simulink model "Model_FC_v16_Edit_for_Full_Scale_Fuel_Cell_GAS"  (R2018a)
settings: Solver=VariableStepAuto  StartTime=0  StopTime=inf  FixedStep=0.01  RelTol=1e-3  EnableMultiTasking=on
undefined symbols (not defined in the file): sigbuilder_block
libraries: fl_lib x8, simulink x6, nesl_utility x4, autolibdcdc x1, powerlib x1
(part 3 of 3)

== system Model_FC_v16_Edit_for_Full_Scale_Fuel_Cell_GAS/Load ==
  note: This Block models the Load Profile as dictated by the ship Resistance in the River Nile
  Signal : Inport
  Bus Selector : BusSelector  OutputSignals=Cell Output Voltage (V),Number Of Cells
  Current from Load profile of one day : Subsystem  Tag=STV Subsys  LoadFcn=sigbuilder_block('load');  StartFcn=sigbuilder_block('start');  StopFcn=sigbuilder_block('stop');  ClipboardFcn=sigbuilder_block('clipboard');  mask(Sigbuilder block){tuvar=[0:10]}
      mask help: Simulink:masks:SigbuilderBlock_MD
      mask init:
      | if ~strcmp(get_param(bdroot(gcbh),'SimulationStatus'),'stopped') tuvar = sigbuilder_block('maskInit'); end
      settings: CopyFcn=sigbuilder_block('copy');  DeleteFcn=sigbuilder_block('delete');  ModelCloseFcn=sigbuilder_block('modelClose');  PreSaveFcn=sigbuilder_block('preSave');  PauseFcn=sigbuilder_block('pause');  ContinueFcn=sigbuilder_block('continue');  NameChangeFcn=sigbuilder_block('namechange');  OpenFcn=sigbuilder_block('open',[403.5 117 550.5 359.25 ]);  CloseFcn=sigbuilder_block('close');
      mask Display: plot(0, 0, 100, 100,[2, 2, 32, 32, 2], [68, 8, 8, 68, 68],[32, 2], [38, 38], [32, 19, 2],[53, 60, 44], [32, 17, 17, 2],[16, 16, 31, 31]);txt = getActiveGroup(gcbh);text(2, 100, txt,'verticalAlignment', 'top');
  Product : Product
  Terminator : Terminator
  Load Profile Current : Outport
  Total Output Voltage (V) : Outport  Port=2
  wires:
  Signal/1 -> Bus Selector/1
  Bus Selector/1 -> Product/1  "<Cell Output Voltage (V)>"
  Product/1 -> Total Output Voltage (V)/1  "Total Output Voltage (V)"
  Current from Load profile of one day/2(Signal 2) -> Load Profile Current/1  "Current from Load profile (Alex to Aswan)"
  Bus Selector/2 -> Product/2  "<Number Of Cells>"
  Current from Load profile of one day/1(Signal 1) -> Terminator/1  "Current from Load profile (Alex to Aswan)"

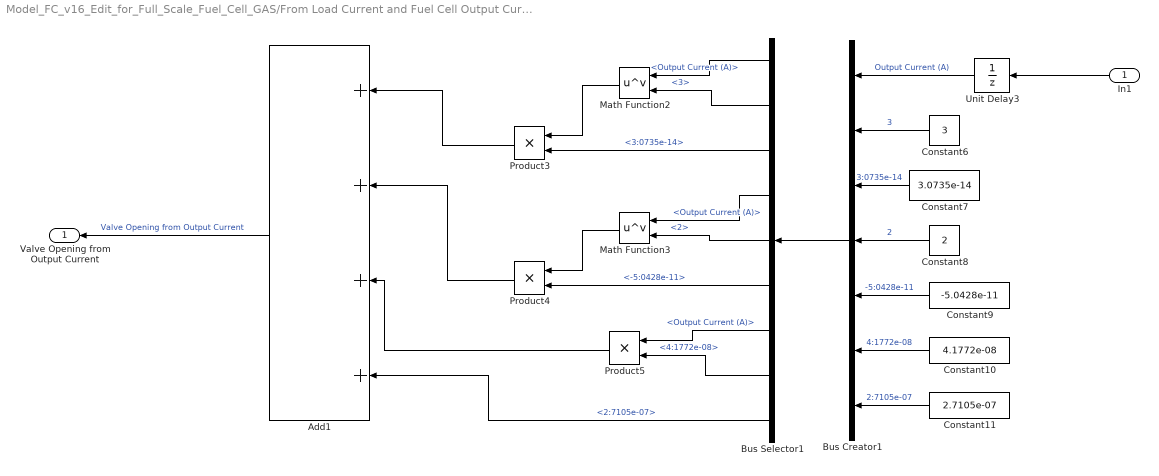
== system Model_FC_v16_Edit_for_Full_Scale_Fuel_Cell_GAS/From Load Current and Fuel Cell Output Current (A) to Valve Restriction Area (m^2)/Subsystem ==
  In1 : Inport
  Add1 : Sum  Inputs=4
  Bus Creator1 : BusCreator  Inputs=7
  Bus Selector1 : BusSelector  OutputSignals=Output Current (A),3,3:0735e-14,Output Current (A),2,-5:0428e-11,Output Current (A),4:1772e-08,2:7105e-07
  Constant10 : Constant  Value=4.1772e-08
  Constant11 : Constant  Value=2.7105e-07
  Constant6 : Constant  Value=3
  Constant7 : Constant  Value=3.0735e-14
  Constant8 : Constant  Value=2
  Constant9 : Constant  Value=-5.0428e-11
  Math Function2 : Math  Operator=pow  SaturateOnIntegerOverflow=on
  Math Function3 : Math  Operator=pow  SaturateOnIntegerOverflow=on
  Product3 : Product
  Product4 : Product
  Product5 : Product
  Unit Delay3 : UnitDelay  SampleTime=-1
  Valve Opening from Output Current : Outport
  wires:
  Product3/1 -> Add1/1
  Constant9/1 -> Bus Creator1/5  "-5:0428e-11"
  Constant11/1 -> Bus Creator1/7  "2:7105e-07"
  Constant8/1 -> Bus Creator1/4  "2"
  Constant6/1 -> Bus Creator1/2  "3"
  Bus Selector1/5 -> Math Function3/2  "<2>"
  Constant10/1 -> Bus Creator1/6  "4:1772e-08"
  In1/1 -> Unit Delay3/1
  Math Function2/1 -> Product3/1
  Math Function3/1 -> Product4/1
  Bus Selector1/3 -> Product3/2  "<3:0735e-14>"
  Bus Selector1/9 -> Add1/4  "<2:7105e-07>"
  Bus Selector1/2 -> Math Function2/2  "<3>"
  Bus Creator1/1 -> Bus Selector1/1
  Bus Selector1/6 -> Product4/2  "<-5:0428e-11>"
  Bus Selector1/8 -> Product5/2  "<4:1772e-08>"
  Bus Selector1/4 -> Math Function3/1  "<Output Current (A)>"
  Product4/1 -> Add1/2
  Product5/1 -> Add1/3
  Constant7/1 -> Bus Creator1/3  "3:0735e-14"
  Unit Delay3/1 -> Bus Creator1/1  "Output Current (A)"
  Bus Selector1/7 -> Product5/1  "<Output Current (A)>"
  Bus Selector1/1 -> Math Function2/1  "<Output Current (A)>"
  Add1/1 -> Valve Opening from Output Current/1  "Valve Opening from Output Current"

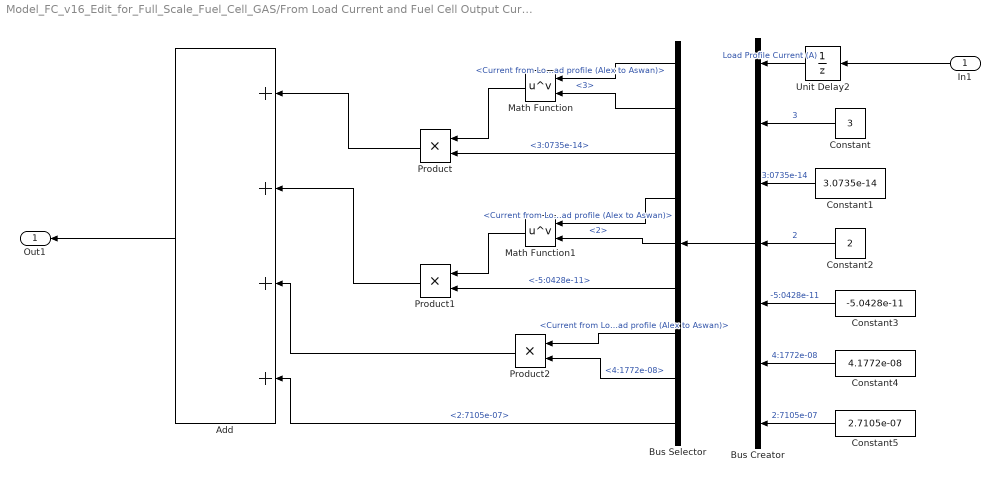
== system Model_FC_v16_Edit_for_Full_Scale_Fuel_Cell_GAS/From Load Current and Fuel Cell Output Current (A) to Valve Restriction Area (m^2)/Subsystem1 ==
  In1 : Inport
  Add : Sum  Inputs=4
  Bus Creator : BusCreator  Inputs=7
  Bus Selector : BusSelector  OutputSignals=Load Profile Current (A).Current from Load profile (Alex to Aswan),3,3:0735e-14,Load Profile Current (A).Current from Load profile (Alex to Aswan),2,-5:0428e-11,Load Profile Current (A).Current from Load profile (Alex to Aswan),4:1772e-08,2:7105e-07
  Constant : Constant  Value=3
  Constant1 : Constant  Value=3.0735e-14
  Constant2 : Constant  Value=2
  Constant3 : Constant  Value=-5.0428e-11
  Constant4 : Constant  Value=4.1772e-08
  Constant5 : Constant  Value=2.7105e-07
  Math Function : Math  Operator=pow  SaturateOnIntegerOverflow=on
  Math Function1 : Math  Operator=pow  SaturateOnIntegerOverflow=on
  Product : Product
  Product1 : Product
  Product2 : Product
  Unit Delay2 : UnitDelay  SampleTime=-1
  Out1 : Outport
  wires:
  Bus Selector/2 -> Math Function/2  "<3>"
  Bus Selector/5 -> Math Function1/2  "<2>"
  Product/1 -> Add/1
  Constant/1 -> Bus Creator/2  "3"
  Unit Delay2/1 -> Bus Creator/1  "Load Profile Current (A)"
  Constant5/1 -> Bus Creator/7  "2:7105e-07"
  Constant2/1 -> Bus Creator/4  "2"
  Bus Selector/1 -> Math Function/1  "<Current from Load profile (Alex to Aswan)>"
  Constant3/1 -> Bus Creator/5  "-5:0428e-11"
  Constant4/1 -> Bus Creator/6  "4:1772e-08"
  Bus Selector/7 -> Product2/1  "<Current from Load profile (Alex to Aswan)>"
  Math Function1/1 -> Product1/1
  Bus Selector/9 -> Add/4  "<2:7105e-07>"
  Bus Selector/8 -> Product2/2  "<4:1772e-08>"
  Bus Selector/6 -> Product1/2  "<-5:0428e-11>"
  Constant1/1 -> Bus Creator/3  "3:0735e-14"
  Product1/1 -> Add/2
  Math Function/1 -> Product/1
  Bus Creator/1 -> Bus Selector/1
  Product2/1 -> Add/3
  Bus Selector/3 -> Product/2  "<3:0735e-14>"
  Bus Selector/4 -> Math Function1/1  "<Current from Load profile (Alex to Aswan)>"
  In1/1 -> Unit Delay2/1
  Add/1 -> Out1/1

== system Model_FC_v16_Edit_for_Full_Scale_Fuel_Cell_GAS/Fuel Cell Model/ From Current Density (A//cm^2) To Overvoltages (V) ==
  note: This Block calculates all the Resistances in the Fuel Cell
      | 1-Activation Overvoltage 2- Ohmic Overvoltage 3-Concentration Overvoltage
      | INPUTS: INPUTS: A) Current Density (A/cm^2) INPUTS: A) Current Density (A/cm^2)
      | A) Current Density (A/cm^2) OUTPUTS: A) Ohmic Overvoltage (V) OUTPUTS: A) Concentration Overvoltage (V)
      | B) Temperature (c)
      |
      | OUTPUTS:
      | A) Activation Overvoltage (V)
  Current Density (A/cm^2) : Inport
  Temperature (C) : Inport  Port=2
  Activation Overvoltage : Subsystem
  Concentration Overvoltage : Subsystem
  Ohmic Overvoltage : Subsystem
  Activation Overvoltage (V) : Outport
  Ohmic Overvoltage (V) : Outport  Port=2
  Concentration Overvoltage (V) : Outport  Port=3
  Exchange Current Density (i_0) : Outport  Port=4
  wires:
  Temperature (C)/1 -> Activation Overvoltage/1(Temperature/C1)
  Current Density (A/cm^2)/1 -> Activation Overvoltage/2(Current Density (i)(A/cm^2)), Concentration Overvoltage/1(Current Density (i)1), Ohmic Overvoltage/1(Current Density (i ))
  Ohmic Overvoltage/1(V_Resistive) -> Ohmic Overvoltage (V)/1
  Activation Overvoltage/1(Activation Overvoltage1 (V)) -> Activation Overvoltage (V)/1
  Concentration Overvoltage/1("Concentration Overvoltage1 (V) ") -> Concentration Overvoltage (V)/1
  Activation Overvoltage/2(Exchange Current Density (i_0)) -> Exchange Current Density (i_0)/1

== system Model_FC_v16_Edit_for_Full_Scale_Fuel_Cell_GAS/Fuel Cell Model/Air Flow Rate To Current (A) ==
  note: The function of this block is: To calculate the Air Mass Flow Rate in (kg/s) using the Input Current Density (A/cm^2)
      | Inputs: Outputs:
      | a) Current DEnsity (A/cm^2) A) Air Mass Flow Rate (kg/s)
      | b) Cell Area (cm^2)
      | c) Number of Cells
  Current Density (A/cm^2) : Inport
  Cell Area (cm^2) : Inport  Port=2
  Number Of Cells : Inport  Port=3
  Air Molar Mass (Kg) : Constant  Value=28.9647e-3
  Current (A) : Product
  Divide : Product  Inputs=*/
  From Stack Current (A) To Oxygen Mass Flow Rate(kg/s) : Subsystem
  Oxygen Molar Mass per One Mole of Air (Kg) : Constant  Value=6.72e-3
  Product : Product
  Air Mass Flow Rate (kg/s) : Outport
  wires:
  Current (A)/1 -> From Stack Current (A) To Oxygen Mass Flow Rate(kg/s)/1(Current (A))
  Number Of Cells/1 -> From Stack Current (A) To Oxygen Mass Flow Rate(kg/s)/2(Number Of Cells)
  From Stack Current (A) To Oxygen Mass Flow Rate(kg/s)/1(Oxygen Flow Rate (kg/s)) -> Product/1
  Current Density (A/cm^2)/1 -> Current (A)/1
  Cell Area (cm^2)/1 -> Current (A)/2
  Air Molar Mass (Kg)/1 -> Product/2
  Product/1 -> Divide/1
  Oxygen Molar Mass per One Mole of Air (Kg)/1 -> Divide/2
  Divide/1 -> Air Mass Flow Rate (kg/s)/1  "Air Mass Flow Rate (kg/s)"

== system Model_FC_v16_Edit_for_Full_Scale_Fuel_Cell_GAS/Fuel Cell Model/Current Density A//cm^2 (Polarization Curve) ==
  Demux : Demux  Tag=STV Demux  Outputs=2
  FromWs : FromWorkspace  Tag=STV FromWs  VariableName=tuvar  SampleTime=0
      SigBuilderData=|
      | common.afterFinalStr = 'Extrapolate'
      | common.sampleTime = 0
      | dataSet.timeRange = [0 20]
      | dataSet.name = 'Group 1'
      | sbobj.Groups.Name = 'Group 1'
      | sbobj.Groups.Signals(1).Name = 'Signal 1'
      | sbobj.Groups.Signals(1).XData = [0 0.5 1 20]
      | sbobj.Groups.Signals(1).YData = [0.01 1 1.4 1.4]
      | sbobj.Groups.Signals(2).Name = 'Signal 2'
      | sbobj.Groups.Signals(2).XData = [0 20]
      | sbobj.Groups.Signals(2).YData = [1 1]
      | sbobj.Groups.TimeRange = [0 20]
  Signal 1 : Outport  Tag=STV Outport
  Signal 2 : Outport  Tag=STV Outport  Port=2
  wires:
  Demux/1 -> Signal 1/1
  FromWs/1 -> Demux/1
  Demux/2 -> Signal 2/1

== system Model_FC_v16_Edit_for_Full_Scale_Fuel_Cell_GAS/Fuel Cell Model/From Mass Flow Rates (kg//s) To Current Density (A//cm^2) ==
  note: The function of this block is to convert the input Hydrogen Mass Flow rate (Kg/s) to Current (A) then divide it by the Cell Area (cm^2) to get (Current Density) (A/cm^2)
      | which will be the input of several other blocks.
      | Inputs: a)Hydrogen Mass Flow Rate (kg/s) Outputs: Current Density (A/cm^2)
      | b)Number of Cells
      | c) Cell Area (cm^2)
  Hydrogen Flow Rate (kg/s) : Inport
  Cell Area (cm^2) : Inport  Port=2
  Number Of Cells : Inport  Port=3
  From Current (A) To Current Density (A/cm^2) : Subsystem
  Fuel Mass Flow Rate (kg/s) To Current (A) : Subsystem
  Current Density (A/cm^2) : Outport
  wires:
  Cell Area (cm^2)/1 -> From Current (A) To Current Density (A/cm^2)/2(Cell Area (cm^2))
  Fuel Mass Flow Rate (kg/s) To Current (A)/1(Current (A)) -> From Current (A) To Current Density (A/cm^2)/1(Nominal Current (A))
  Hydrogen Flow Rate (kg/s)/1 -> Fuel Mass Flow Rate (kg/s) To Current (A)/1(Hydrogen Flow Rate (kg/s))
  From Current (A) To Current Density (A/cm^2)/1(Current Density (A/cm^2)) -> Current Density (A/cm^2)/1  "Current density (A/cm^2)"
  Number Of Cells/1 -> Fuel Mass Flow Rate (kg/s) To Current (A)/2(Number Of Cells)  "Number Of Cells"

== system Model_FC_v16_Edit_for_Full_Scale_Fuel_Cell_GAS/Fuel Cell Model/From Pressures (atm) To Nernest Voltage (V) ==
  note: This Block calculates the Partial Pressures of Hydrogen and Oxygen (atm) from their pressures (atm) then uses these values to calculate the Nernest Voltage (V)
      |
      | INPUTS: A) Current Density (i) (A/cm^2) OUTPUTS 1: A) Oxygen Partial Pressure (atm) OUTPUTS 2: A) Nernest Voltage (V)
      | B) Absolute Hydrogen Pressure (atm) B) Water Saturation Pressure (atm)
      | C) Absolute Air Pressure (atm) C) Hydrogen Partial Pressure(atm)
      | D) Temperature (c)
  Current Density (i) : Inport
  Hydrogen Pressure (atm) : Inport  Port=2
  Air Pressure (atm) : Inport  Port=3
  Temperature (C) : Inport  Port=4
  From Absolute Pressure (atm) To Partial Pressures (atm) : Subsystem
  From Partial Pressures (atm) To Nernest Voltage (V) : Subsystem
  Oxygen Partial Pressure : Outport
  Nernest Voltage (V) : Outport  Port=2
  Water Pressure : Outport  Port=3
  wires:
  Temperature (C)/1 -> From Partial Pressures (atm) To Nernest Voltage (V)/4(Temperature/C), From Absolute Pressure (atm) To Partial Pressures (atm)/4(Temperature/C)
  From Absolute Pressure (atm) To Partial Pressures (atm)/1(Hydrogen Partial Pressure (pp_H2)) -> From Partial Pressures (atm) To Nernest Voltage (V)/1(Hydrogen Partial Pressure)
  Hydrogen Pressure (atm)/1 -> From Absolute Pressure (atm) To Partial Pressures (atm)/2(Hydrogen Pressure (P_H2))
  From Partial Pressures (atm) To Nernest Voltage (V)/1(Nernest Voltage1) -> Nernest Voltage (V)/1
  From Absolute Pressure (atm) To Partial Pressures (atm)/2(Oxygen Partial Pressure pp_O2) -> Oxygen Partial Pressure/1, From Partial Pressures (atm) To Nernest Voltage (V)/2(Oxygen Partial Pressure)
  From Absolute Pressure (atm) To Partial Pressures (atm)/3(Water Pressure) -> Water Pressure/1, From Partial Pressures (atm) To Nernest Voltage (V)/3(Water Pressure (P_H2O))
  Current Density (i)/1 -> From Absolute Pressure (atm) To Partial Pressures (atm)/1(Current Density (i ))
  Air Pressure (atm)/1 -> From Absolute Pressure (atm) To Partial Pressures (atm)/3(Air Pressure (P_air))

== system Model_FC_v16_Edit_for_Full_Scale_Fuel_Cell_GAS/Load/Current from Load profile of one day ==
  Demux : Demux  Tag=STV Demux  Outputs=2
  FromWs : FromWorkspace  Tag=STV FromWs  VariableName=tuvar  SampleTime=0
      SigBuilderData=|
      | common.afterFinalStr = 'Extrapolate'
      | common.sampleTime = 0
      | dataSet.timeRange = [0 300]
      | dataSet.name = 'Group 1'
      | sbobj.Groups.Name = 'Group 1'
      | sbobj.Groups.Signals(1).Name = 'Signal 1'
      | sbobj.Groups.Signals(1).XData = [0 2.75 2.75 5.75 5.75 10.98 10.98 24 24 24.6 24.6 27.61 27.61 30.61 30.61 33.73 33.73 36.73 48 48 52.19 52.19 55.19 55.19 59.38 59.38 62.38 72 72 84 84 96 96 108 108 120 120 132 132 144 144 146.76 146.76 147.76 147.76 156 156 168 168 175.76 175.76 176.76 176.76 180 180 192 192 204 204 216 216 216.76 216.76 217.76 217.76 228 228 240 240 244.83 244.83 300]
      | sbobj.Groups.Signals(1).YData = [145.4545455 145.4545455 0.01 0.01 145.4545455 145.4545455 0.01 0.01 195.4545455 195.4545455 486.3636364 486.3636364 0.01 0.01 404.5454545 404.5454545 0.01 0.01 0.01 486.3636364 486.3636364 0.01 0.01 486.3636364 486.3636364 0.01 0.01 0.01 463.6363636 463.6363636 0.01 0.01 463.6363636 463.6363636 0.01 0.01 463.6363636 463.6363636 0.01 0.01 463.6363636 463.6363636 0.01 0.01 463.6363636 463.6363636 0.01 0.01 463.6363636 463.6363636 0.01 0.01 463.6363636 463.6363636 0.01 0.01 463.6363636 463.6363636 0.01 0.01 463.6363636 463.6363636 0.01 0.01 463.6363636 463.6363636 0.01 0.01 463.6363636 463.6363636 0.01 0.01]
      | sbobj.Groups.Signals(2).Name = 'Signal 2'
      | sbobj.Groups.Signals(2).XData = [0 300]
      | sbobj.Groups.Signals(2).YData = [243 243]
      | sbobj.Groups.TimeRange = [0 300]
  Signal 1 : Outport  Tag=STV Outport
  Signal 2 : Outport  Tag=STV Outport  Port=2
  wires:
  Demux/1 -> Signal 1/1
  FromWs/1 -> Demux/1
  Demux/2 -> Signal 2/1

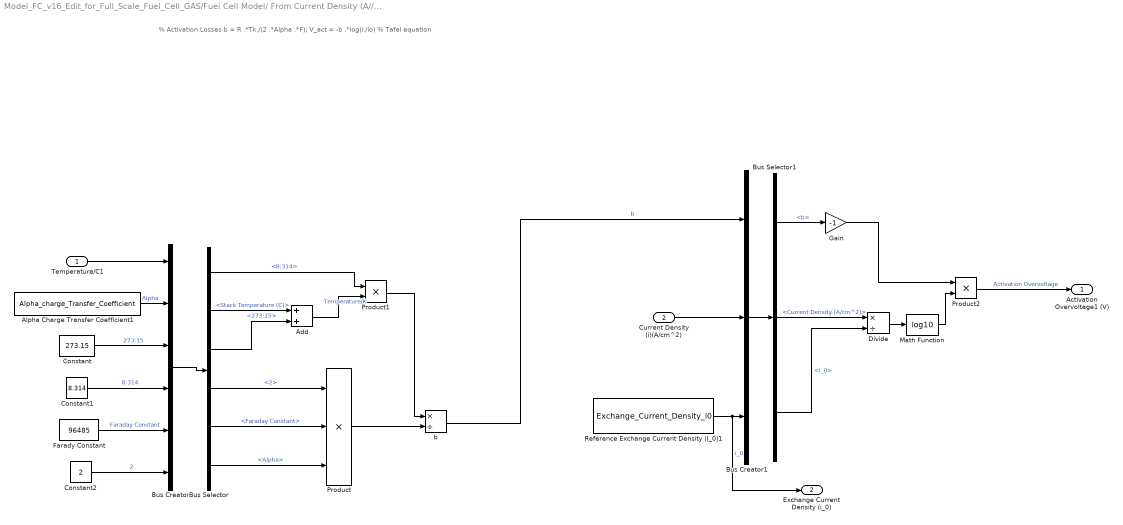
== system Model_FC_v16_Edit_for_Full_Scale_Fuel_Cell_GAS/Fuel Cell Model/ From Current Density (A//cm^2) To Overvoltages (V)/Activation Overvoltage ==
  note: % Activation Losses
      | b = R .*Tk./(2 .*Alpha .*F);
      | V_act = -b .*log(i./io) % Tafel equation
  Temperature/C1 : Inport
  Current Density (i)(A/cm^2) : Inport  Port=2
  Add : Sum
  Alpha Charge Transfer Coefficient1 : Constant  Value=Alpha_charge_Transfer_Coefficient
  Bus Creator : BusCreator  Inputs=6
  Bus Creator1 : BusCreator  Inputs=3
  Bus Selector : BusSelector  OutputSignals=8:314,Stack Temperature (C),273:15,2,Faraday Constant,Alpha
  Bus Selector1 : BusSelector  OutputSignals=b,Current Density (A/cm^2),i_0
  Constant : Constant  Value=273.15
  Constant1 : Constant  Value=8.314
  Constant2 : Constant  Value=2
  Divide : Product  Inputs=*/
  Farady Constant : Constant  Value=96485
  Gain : Gain  Gain=-1
  Math Function : Math  Operator=log10  SaturateOnIntegerOverflow=on
  Product : Product  Inputs=3
  Product1 : Product
  Product2 : Product
  Reference Exchange Current Density (I_0)1 : Constant  Value=Exchange_Current_Density_i0
  b : Product  Inputs=*/
  Activation Overvoltage1 (V) : Outport
  Exchange Current Density (i_0) : Outport  Port=2
  wires:
  Alpha Charge Transfer Coefficient1/1 -> Bus Creator/2  "Alpha"
  Temperature/C1/1 -> Bus Creator/1
  Current Density (i)(A/cm^2)/1 -> Bus Creator1/2
  Reference Exchange Current Density (I_0)1/1 -> Bus Creator1/3, Exchange Current Density (i_0)/1  "i_0"
  Product2/1 -> Activation Overvoltage1 (V)/1  "Activation Overvoltage"
  Bus Creator/1 -> Bus Selector/1
  Constant/1 -> Bus Creator/3  "273:15"
  Constant1/1 -> Bus Creator/4  "8:314"
  Farady Constant/1 -> Bus Creator/5  "Faraday Constant"
  Constant2/1 -> Bus Creator/6  "2"
  Bus Selector/4 -> Product/1  "<2>"
  Bus Selector/5 -> Product/2  "<Faraday Constant>"
  Bus Selector/6 -> Product/3  "<Alpha>"
  Product/1 -> b/2
  Bus Selector/1 -> Product1/1  "<8:314>"
  Bus Selector/2 -> Add/1  "<Stack Temperature (C)>"
  Bus Selector/3 -> Add/2  "<273:15>"
  Add/1 -> Product1/2  "Temperature/K"
  Product1/1 -> b/1
  b/1 -> Bus Creator1/1  "b"
  Bus Creator1/1 -> Bus Selector1/1
  Bus Selector1/1 -> Gain/1  "<b>"
  Bus Selector1/2 -> Divide/1  "<Current Density (A/cm^2)>"
  Bus Selector1/3 -> Divide/2  "<i_0>"
  Gain/1 -> Product2/1
  Divide/1 -> Math Function/1
  Math Function/1 -> Product2/2

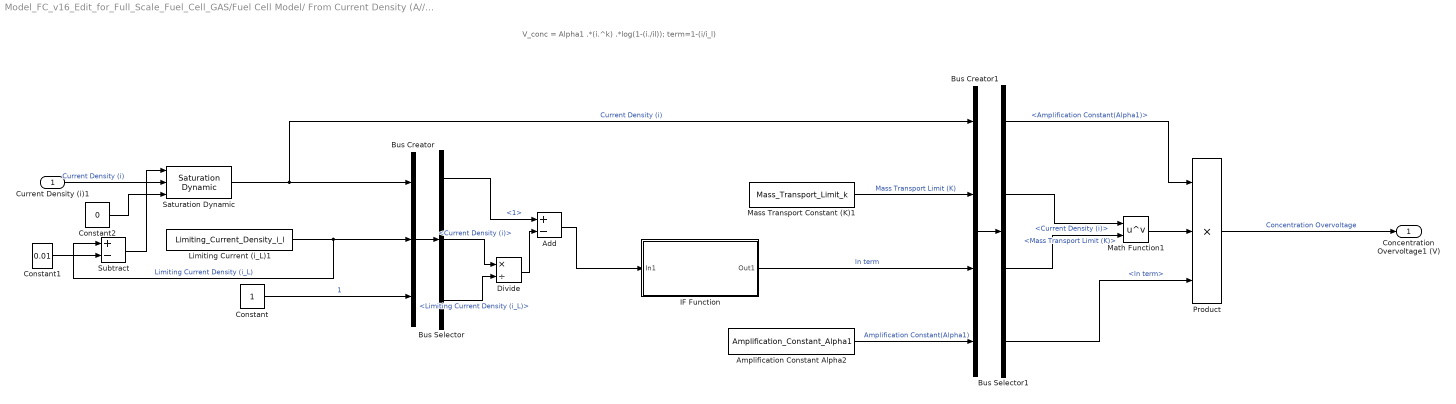
== system Model_FC_v16_Edit_for_Full_Scale_Fuel_Cell_GAS/Fuel Cell Model/ From Current Density (A//cm^2) To Overvoltages (V)/Concentration Overvoltage ==
  note: V_conc = Alpha1 .*(i.^k) .*log(1-(i./il));
      | term=1-(i/i_l)
  Current Density (i)1 : Inport
  Add : Sum  Inputs=+-
  Amplification Constant Alpha2 : Constant  Value=Amplification_Constant_Alpha1
  Bus Creator : BusCreator  Inputs=3
  Bus Creator1 : BusCreator  Inputs=4
  Bus Selector : BusSelector  OutputSignals=1,Current Density (i),Limiting Current Density (i_L)
  Bus Selector1 : BusSelector  OutputSignals=Amplification Constant(Alpha1),Current Density (i),Mass Transport Limit (K),ln term
  Constant : Constant
  Constant1 : Constant  Value=0.01
  Constant2 : Constant  Value=0
  Divide : Product  Inputs=*/
  IF Function : Subsystem
  Limiting Current (i_L)1 : Constant  Value=Limiting_Current_Density_i_l
  Mass Transport Constant (K)1 : Constant  Value=Mass_Transport_Limit_k
  Math Function1 : Math  Operator=pow  SaturateOnIntegerOverflow=on
  Product : Product  Inputs=3
  Saturation Dynamic : simulink/Discontinuities/Saturation Dynamic  OutMin=[]  OutMax=[]  OutDataTypeStr=Inherit: Same as second input  OutDataType=fixdt(1, 16)  OutScaling=2^-10  DoSatur=off
  Subtract : Sum  Inputs=+-
  "Concentration Overvoltage1 (V) " : Outport
  wires:
  Bus Creator/1 -> Bus Selector/1
  Limiting Current (i_L)1/1 -> Subtract/1, Bus Creator/2  "Limiting Current Density (i_L)"
  Saturation Dynamic/1 -> Bus Creator1/1, Bus Creator/1  "Current Density (i)"
  Mass Transport Constant (K)1/1 -> Bus Creator1/2  "Mass Transport Limit (K)"
  Amplification Constant Alpha2/1 -> Bus Creator1/4  "Amplification Constant(Alpha1)"
  Product/1 -> "Concentration Overvoltage1 (V) "/1  "Concentration Overvoltage"
  Constant/1 -> Bus Creator/3  "1"
  Bus Selector/1 -> Add/1  "<1>"
  Bus Selector/2 -> Divide/1  "<Current Density (i)>"
  Bus Selector/3 -> Divide/2  "<Limiting Current Density (i_L)>"
  Divide/1 -> Add/2
  Add/1 -> IF Function/1(In1)
  IF Function/1(Out1) -> Bus Creator1/3  "ln term"
  Bus Creator1/1 -> Bus Selector1/1
  Bus Selector1/1 -> Product/1  "<Amplification Constant(Alpha1)>"
  Bus Selector1/2 -> Math Function1/1  "<Current Density (i)>"
  Bus Selector1/3 -> Math Function1/2  "<Mass Transport Limit (K)>"
  Bus Selector1/4 -> Product/3  "<ln term>"
  Math Function1/1 -> Product/2
  Current Density (i)1/1 -> Saturation Dynamic/2  "Current Density (i)"
  Constant1/1 -> Subtract/2
  Subtract/1 -> Saturation Dynamic/1
  Constant2/1 -> Saturation Dynamic/3

== system Model_FC_v16_Edit_for_Full_Scale_Fuel_Cell_GAS/Fuel Cell Model/ From Current Density (A//cm^2) To Overvoltages (V)/Ohmic Overvoltage ==
  Current Density (i ) : Inport
  Constant : Constant  Value=-1
  Internal Resistance (r) : Constant  Value=Internal_Resistance_r
  V_Resistive1 : Product  Inputs=3
  V_Resistive : Outport
  wires:
  Constant/1 -> V_Resistive1/3
  Internal Resistance (r)/1 -> V_Resistive1/2
  Current Density (i )/1 -> V_Resistive1/1
  V_Resistive1/1 -> V_Resistive/1  "Ohmic Overvoltage (V)"

== system Model_FC_v16_Edit_for_Full_Scale_Fuel_Cell_GAS/Fuel Cell Model/Air Flow Rate To Current (A)/From Stack Current (A) To Oxygen Mass Flow Rate(kg//s) ==
  Current (A) : Inport
  Number Of Cells : Inport  Port=2
  Divide : Product  Inputs=*/
  F : Constant  Value=96487
  Oxygen Molar Mass (Kg/mol) : Constant  Value=32e-3
  Product : Product
  Product1 : Product
  Product2 : Product
  c : Constant  Value=4
  Oxygen Flow Rate (kg/s) : Outport
  wires:
  F/1 -> Product1/1
  Current (A)/1 -> Product/1
  Product/1 -> Divide/1
  Oxygen Molar Mass (Kg/mol)/1 -> Product2/2
  c/1 -> Product1/2
  Divide/1 -> Product2/1
  Product1/1 -> Divide/2
  Product2/1 -> Oxygen Flow Rate (kg/s)/1
  Number Of Cells/1 -> Product/2

== system Model_FC_v16_Edit_for_Full_Scale_Fuel_Cell_GAS/Fuel Cell Model/From Mass Flow Rates (kg//s) To Current Density (A//cm^2)/From Current (A) To Current Density (A//cm^2) ==
  note: i=I/A
      | where i=Current Density (A/cm^2)
      | I= Current (A)
      | A=Cell Area (cm^2)
  Nominal Current (A) : Inport
  Cell Area (cm^2) : Inport  Port=2
  Divide : Product  Inputs=*/
  Current Density (A/cm^2) : Outport
  wires:
  Nominal Current (A)/1 -> Divide/1
  Cell Area (cm^2)/1 -> Divide/2
  Divide/1 -> Current Density (A/cm^2)/1

== system Model_FC_v16_Edit_for_Full_Scale_Fuel_Cell_GAS/Fuel Cell Model/From Mass Flow Rates (kg//s) To Current Density (A//cm^2)/Fuel Mass Flow Rate (kg//s) To Current (A) ==
  note: This block calculates the output Current (A) from the Hydrogen Mass Flow Rate (kg/s)
      | I=Hydrogen Mass Flow Rate (kg/s)*2*F/(M_H2*n)
      | where: I=Current (A)
      | F=Faraday Constant=96487 C/mol
      | M_H2=hydrogen molar mass=2.016*10^-3 kg/mol
      | n=Number of Cells
  Hydrogen Flow Rate (kg/s) : Inport
  Number Of Cells : Inport  Port=2
  Constant1 : Constant  Value=2
  Divide : Product  Inputs=*/
  F : Constant  Value=96487
  Hydrogen Molar Mass : Constant  Value=2.016e-3
  Product : Product
  Product1 : Product
  Product2 : Product
  Current (A) : Outport
  wires:
  F/1 -> Product1/2
  Constant1/1 -> Product1/1
  Product1/1 -> Product/2
  Product/1 -> Divide/1
  Hydrogen Molar Mass/1 -> Product2/1
  Number Of Cells/1 -> Product2/2
  Product2/1 -> Divide/2
  Divide/1 -> Current (A)/1
  Hydrogen Flow Rate (kg/s)/1 -> Product/1

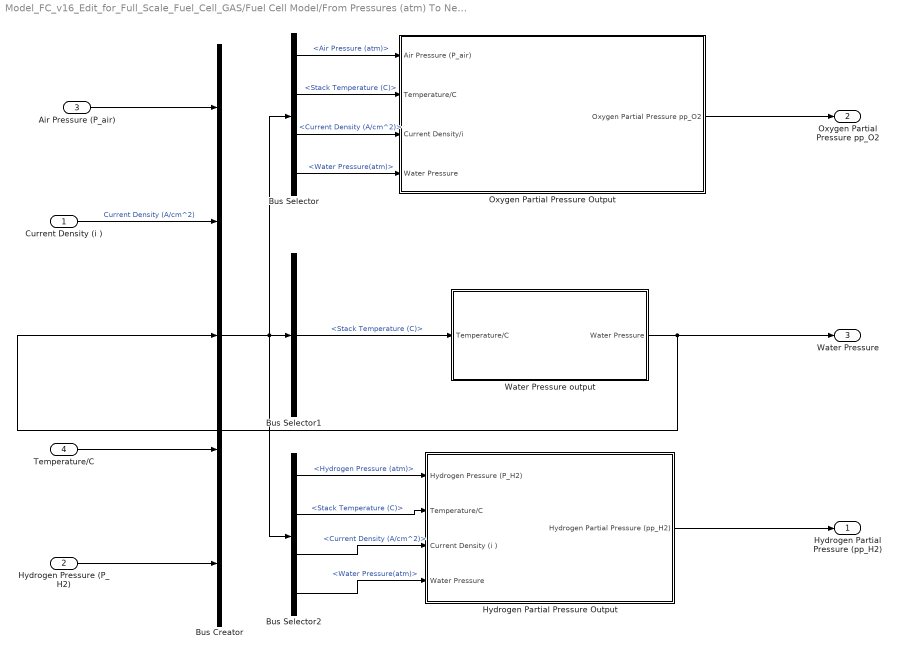
== system Model_FC_v16_Edit_for_Full_Scale_Fuel_Cell_GAS/Fuel Cell Model/From Pressures (atm) To Nernest Voltage (V)/From Absolute Pressure (atm) To Partial Pressures (atm) ==
  Current Density (i ) : Inport
  Hydrogen Pressure (P_H2) : Inport  Port=2
  Air Pressure (P_air) : Inport  Port=3
  Temperature/C : Inport  Port=4
  Bus Creator : BusCreator  Inputs=5
  Bus Selector : BusSelector  OutputSignals=Air Pressure (atm),Stack Temperature (C),Current Density (A/cm^2),Water Pressure(atm)
  Bus Selector1 : BusSelector  OutputSignals=Stack Temperature (C)
  Bus Selector2 : BusSelector  OutputSignals=Hydrogen Pressure (atm),Stack Temperature (C),Current Density (A/cm^2),Water Pressure(atm)
  Hydrogen Partial Pressure Output : Subsystem
  Oxygen Partial Pressure Output : Subsystem
  Water Pressure output : Subsystem
  Hydrogen Partial Pressure (pp_H2) : Outport
  Oxygen Partial Pressure pp_O2 : Outport  Port=2
  Water Pressure : Outport  Port=3
  wires:
  Water Pressure output/1(Water Pressure) -> Water Pressure/1, Bus Creator/3
  Air Pressure (P_air)/1 -> Bus Creator/1
  Oxygen Partial Pressure Output/1(Oxygen Partial Pressure pp_O2) -> Oxygen Partial Pressure pp_O2/1
  Hydrogen Partial Pressure Output/1(Hydrogen Partial Pressure (pp_H2)) -> Hydrogen Partial Pressure (pp_H2)/1
  Current Density (i )/1 -> Bus Creator/2  "Current Density (A/cm^2)"
  Temperature/C/1 -> Bus Creator/4
  Hydrogen Pressure (P_H2)/1 -> Bus Creator/5
  Bus Creator/1 -> Bus Selector2/1, Bus Selector/1, Bus Selector1/1
  Bus Selector/1 -> Oxygen Partial Pressure Output/1(Air Pressure (P_air))  "<Air Pressure (atm)>"
  Bus Selector/2 -> Oxygen Partial Pressure Output/2(Temperature/C)  "<Stack Temperature (C)>"
  Bus Selector/3 -> Oxygen Partial Pressure Output/3(Current Density/i)  "<Current Density (A/cm^2)>"
  Bus Selector/4 -> Oxygen Partial Pressure Output/4(Water Pressure)  "<Water Pressure(atm)>"
  Bus Selector1/1 -> Water Pressure output/1(Temperature/C)  "<Stack Temperature (C)>"
  Bus Selector2/1 -> Hydrogen Partial Pressure Output/1(Hydrogen Pressure (P_H2))  "<Hydrogen Pressure (atm)>"
  Bus Selector2/2 -> Hydrogen Partial Pressure Output/2(Temperature/C)  "<Stack Temperature (C)>"
  Bus Selector2/3 -> Hydrogen Partial Pressure Output/3(Current Density (i ))  "<Current Density (A/cm^2)>"
  Bus Selector2/4 -> Hydrogen Partial Pressure Output/4(Water Pressure)  "<Water Pressure(atm)>"

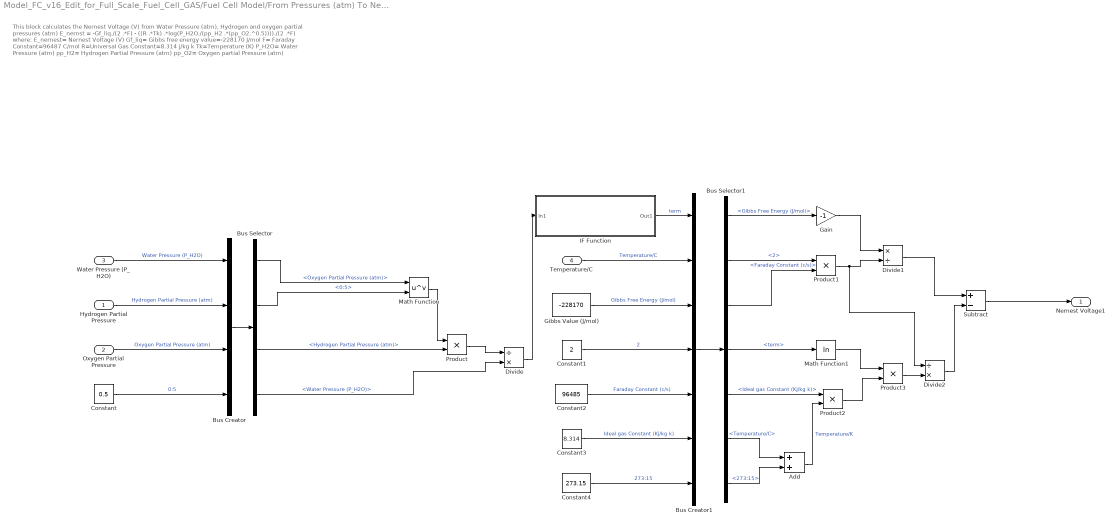
== system Model_FC_v16_Edit_for_Full_Scale_Fuel_Cell_GAS/Fuel Cell Model/From Pressures (atm) To Nernest Voltage (V)/From Partial Pressures (atm) To Nernest Voltage (V) ==
  note: This block calculates the Nernest Voltage (V) from Water Pressure (atm), Hydrogen and oxygen partial pressures (atm)
      | E_nernst = -Gf_liq./(2 .*F) - ((R .*Tk) .*log(P_H2O./(pp_H2 .*(pp_O2.^0.5))))./(2 .*F)
      | where: E_nernest= Nernest Voltage (V)
      | Gf_liq= Gibbs free energy value=-228170 J/mol
      | F= Faraday Constant=96487 C/mol
      | R=Universal Gas Constant=8.314 j/kg k
      | Tk=Temperature (K)
      | P_H2O= Water Pressure (atm)
      | pp_H2= Hydrogen Partial Pressure (atm)
      | pp_O2= Oxygen partial Pressure (atm)
  Hydrogen Partial Pressure : Inport
  Oxygen Partial Pressure : Inport  Port=2
  Water Pressure (P_H2O) : Inport  Port=3
  Temperature/C : Inport  Port=4
  Add : Sum
  Bus Creator : BusCreator  Inputs=4
  Bus Creator1 : BusCreator  Inputs=7
  Bus Selector : BusSelector  OutputSignals=Oxygen Partial Pressure (atm),0:5,Hydrogen Partial Pressure (atm),Water Pressure (P_H2O)
  Bus Selector1 : BusSelector  OutputSignals=Gibbs Free Energy (J/mol),2,Faraday Constant (c/s),term,Ideal gas Constant (Kj/kg k),Temperature/C,273:15
  Constant : Constant  Value=0.5
  Constant1 : Constant  Value=2
  Constant2 : Constant  Value=96485
  Constant3 : Constant  Value=8.314
  Constant4 : Constant  Value=273.15
  Divide : Product  Inputs=/*
  Divide1 : Product  Inputs=*/
  Divide2 : Product  Inputs=/*
  Gain : Gain  Gain=-1
  Gibbs Value (J/mol) : Constant  Value=-228170
  IF Function : Subsystem
  Math Function : Math  Operator=pow  SaturateOnIntegerOverflow=on
  Math Function1 : Math  Operator=log  SaturateOnIntegerOverflow=on
  Product{,1..3} (4 alike) : Product
  Subtract : Sum  Inputs=+-
  Nernest Voltage1 : Outport
  wires:
  Gibbs Value (J/mol)/1 -> Bus Creator1/3  "Gibbs Free Energy (J/mol)"
  Oxygen Partial Pressure/1 -> Bus Creator/3  "Oxygen Partial Pressure (atm)"
  Water Pressure (P_H2O)/1 -> Bus Creator/1  "Water Pressure (P_H2O)"
  Hydrogen Partial Pressure/1 -> Bus Creator/2  "Hydrogen Partial Pressure (atm)"
  Temperature/C/1 -> Bus Creator1/2  "Temperature/C"
  Bus Creator/1 -> Bus Selector/1
  Bus Selector/2 -> Math Function/2  "<0:5>"
  Constant/1 -> Bus Creator/4  "0:5"
  Bus Selector/1 -> Math Function/1  "<Oxygen Partial Pressure (atm)>"
  Bus Selector/3 -> Product/2  "<Hydrogen Partial Pressure (atm)>"
  Math Function/1 -> Product/1
  Bus Selector/4 -> Divide/2  "<Water Pressure (P_H2O)>"
  Product/1 -> Divide/1
  Divide/1 -> IF Function/1(In1)
  IF Function/1(Out1) -> Bus Creator1/1  "term"
  Bus Creator1/1 -> Bus Selector1/1
  Constant1/1 -> Bus Creator1/4  "2"
  Constant2/1 -> Bus Creator1/5  "Faraday Constant (c/s)"
  Bus Selector1/1 -> Gain/1  "<Gibbs Free Energy (J/mol)>"
  Gain/1 -> Divide1/1
  Bus Selector1/2 -> Product1/1  "<2>"
  Bus Selector1/3 -> Product1/2  "<Faraday Constant (c/s)>"
  Product1/1 -> Divide2/1, Divide1/2
  Divide1/1 -> Subtract/1
  Bus Selector1/4 -> Math Function1/1  "<term>"
  Math Function1/1 -> Product3/1
  Constant3/1 -> Bus Creator1/6  "Ideal gas Constant (Kj/kg k)"
  Constant4/1 -> Bus Creator1/7  "273:15"
  Bus Selector1/5 -> Product2/1  "<Ideal gas Constant (Kj/kg k)>"
  Bus Selector1/6 -> Add/1  "<Temperature/C>"
  Bus Selector1/7 -> Add/2  "<273:15>"
  Add/1 -> Product2/2  "Temperature/K"
  Product2/1 -> Product3/2
  Product3/1 -> Divide2/2
  Divide2/1 -> Subtract/2
  Subtract/1 -> Nernest Voltage1/1

== system Model_FC_v16_Edit_for_Full_Scale_Fuel_Cell_GAS/Fuel Cell Model/ From Current Density (A//cm^2) To Overvoltages (V)/Concentration Overvoltage/IF Function ==
  In1 : Inport
  Compare To Zero : simulink/Logic and Bit Operations/Compare To Zero  relop=<=  OutDataTypeStr=boolean
  If : If  IfExpression=u1 == 0
  If Action Subsystem : Subsystem  TreatAsAtomicUnit=on
  If Action Subsystem1 : Subsystem  TreatAsAtomicUnit=on
  Merge : Merge  InitialOutput=1
  Out1 : Outport
  wires:
  If Action Subsystem1/1(Out1) -> Merge/2
  Compare To Zero/1 -> If/1
  Merge/1 -> Out1/1
  In1/1 -> If Action Subsystem/1(In1), Compare To Zero/1
  If/2 -> If Action Subsystem1/Action
  If Action Subsystem/1(Out1) -> Merge/1
  If/1 -> If Action Subsystem/Action

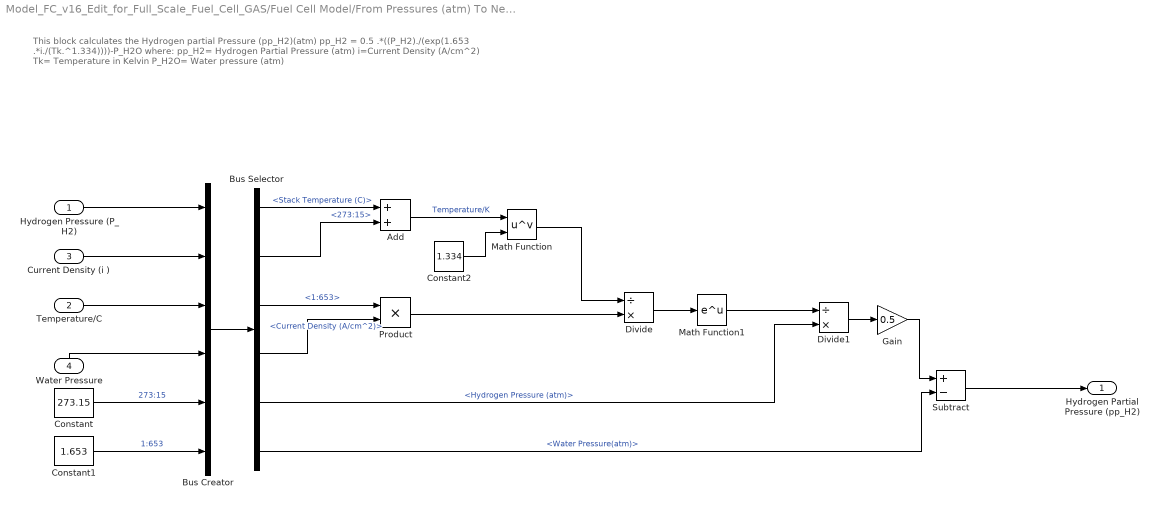
== system Model_FC_v16_Edit_for_Full_Scale_Fuel_Cell_GAS/Fuel Cell Model/From Pressures (atm) To Nernest Voltage (V)/From Absolute Pressure (atm) To Partial Pressures (atm)/Hydrogen Partial Pressure Output ==
  note: This block calculates the Hydrogen partial Pressure (pp_H2)(atm)
      | pp_H2 = 0.5 .*((P_H2)./(exp(1.653 .*i./(Tk.^1.334))))-P_H2O
      | where: pp_H2= Hydrogen Partial Pressure (atm)
      | i=Current Density (A/cm^2)
      | Tk= Temperature in Kelvin
      | P_H2O= Water pressure (atm)
  Hydrogen Pressure (P_H2) : Inport
  Temperature/C : Inport  Port=2
  Current Density (i ) : Inport  Port=3
  Water Pressure : Inport  Port=4
  Add : Sum
  Bus Creator : BusCreator  Inputs=6
  Bus Selector : BusSelector  OutputSignals=Stack Temperature (C),273:15,1:653,Current Density (A/cm^2),Hydrogen Pressure (atm),Water Pressure(atm)
  Constant : Constant  Value=273.15
  Constant1 : Constant  Value=1.653
  Constant2 : Constant  Value=1.334
  Divide : Product  Inputs=/*
  Divide1 : Product  Inputs=/*
  Gain : Gain  Gain=0.5
  Math Function : Math  Operator=pow  SaturateOnIntegerOverflow=on
  Math Function1 : Math  SaturateOnIntegerOverflow=on
  Product : Product
  Subtract : Sum  Inputs=+-
  Hydrogen Partial Pressure (pp_H2) : Outport
  wires:
  Water Pressure/1 -> Bus Creator/4
  Temperature/C/1 -> Bus Creator/3
  Current Density (i )/1 -> Bus Creator/2
  Hydrogen Pressure (P_H2)/1 -> Bus Creator/1
  Bus Creator/1 -> Bus Selector/1
  Bus Selector/5 -> Divide1/2  "<Hydrogen Pressure (atm)>"
  Bus Selector/1 -> Add/1  "<Stack Temperature (C)>"
  Constant/1 -> Bus Creator/5  "273:15"
  Add/1 -> Math Function/1  "Temperature/K"
  Constant1/1 -> Bus Creator/6  "1:653"
  Bus Selector/2 -> Add/2  "<273:15>"
  Bus Selector/3 -> Product/1  "<1:653>"
  Bus Selector/4 -> Product/2  "<Current Density (A/cm^2)>"
  Product/1 -> Divide/2
  Divide/1 -> Math Function1/1
  Constant2/1 -> Math Function/2
  Math Function/1 -> Divide/1
  Math Function1/1 -> Divide1/1
  Divide1/1 -> Gain/1
  Bus Selector/6 -> Subtract/2  "<Water Pressure(atm)>"
  Subtract/1 -> Hydrogen Partial Pressure (pp_H2)/1
  Gain/1 -> Subtract/1

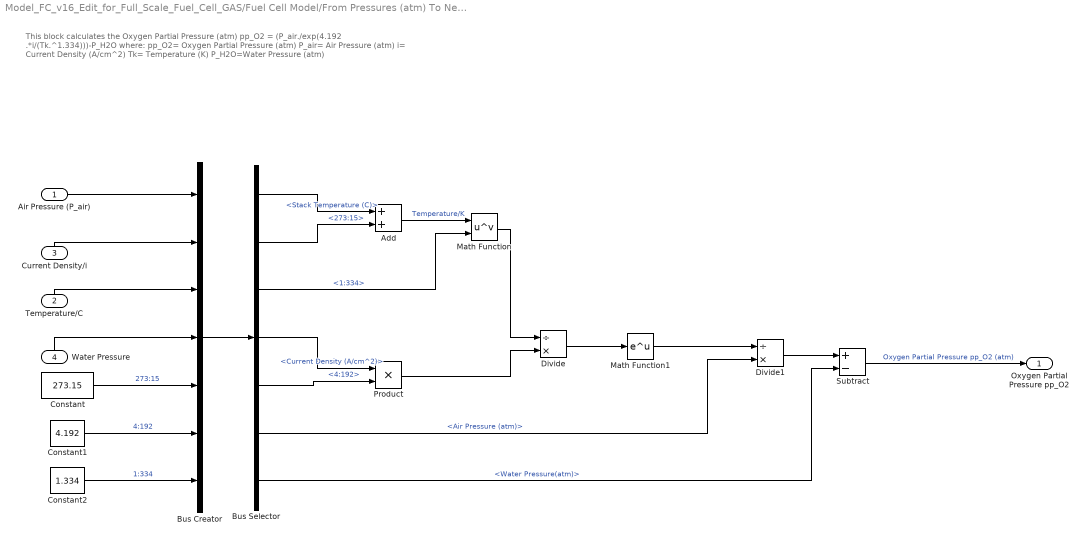
== system Model_FC_v16_Edit_for_Full_Scale_Fuel_Cell_GAS/Fuel Cell Model/From Pressures (atm) To Nernest Voltage (V)/From Absolute Pressure (atm) To Partial Pressures (atm)/Oxygen Partial Pressure Output ==
  note: This block calculates the Oxygen Partial Pressure (atm)
      | pp_O2 = (P_air./exp(4.192 .*i/(Tk.^1.334)))-P_H2O
      |
      | where: pp_O2= Oxygen Partial Pressure (atm)
      | P_air= Air Pressure (atm)
      | i= Current Density (A/cm^2)
      | Tk= Temperature (K)
      | P_H2O=Water Pressure (atm)
  Air Pressure (P_air) : Inport
  Temperature/C : Inport  Port=2
  Current Density/i : Inport  Port=3
  Water Pressure : Inport  Port=4
  Add : Sum
  Bus Creator : BusCreator  Inputs=7
  Bus Selector : BusSelector  OutputSignals=Stack Temperature (C),273:15,1:334,Current Density (A/cm^2),4:192,Air Pressure (atm),Water Pressure(atm)
  Constant : Constant  Value=273.15
  Constant1 : Constant  Value=4.192
  Constant2 : Constant  Value=1.334
  Divide : Product  Inputs=/*
  Divide1 : Product  Inputs=/*
  Math Function : Math  Operator=pow  SaturateOnIntegerOverflow=on
  Math Function1 : Math  SaturateOnIntegerOverflow=on
  Product : Product
  Subtract : Sum  Inputs=+-
  Oxygen Partial Pressure pp_O2 : Outport
  wires:
  Current Density/i/1 -> Bus Creator/2
  Water Pressure/1 -> Bus Creator/4
  Temperature/C/1 -> Bus Creator/3
  Air Pressure (P_air)/1 -> Bus Creator/1
  Constant/1 -> Bus Creator/5  "273:15"
  Constant1/1 -> Bus Creator/6  "4:192"
  Constant2/1 -> Bus Creator/7  "1:334"
  Bus Creator/1 -> Bus Selector/1
  Bus Selector/1 -> Add/1  "<Stack Temperature (C)>"
  Bus Selector/2 -> Add/2  "<273:15>"
  Add/1 -> Math Function/1  "Temperature/K"
  Bus Selector/3 -> Math Function/2  "<1:334>"
  Bus Selector/4 -> Product/1  "<Current Density (A/cm^2)>"
  Bus Selector/5 -> Product/2  "<4:192>"
  Product/1 -> Divide/2
  Math Function/1 -> Divide/1
  Divide/1 -> Math Function1/1
  Math Function1/1 -> Divide1/1
  Bus Selector/6 -> Divide1/2  "<Air Pressure (atm)>"
  Divide1/1 -> Subtract/1
  Bus Selector/7 -> Subtract/2  "<Water Pressure(atm)>"
  Subtract/1 -> Oxygen Partial Pressure pp_O2/1  "Oxygen Partial Pressure pp_O2 (atm)"

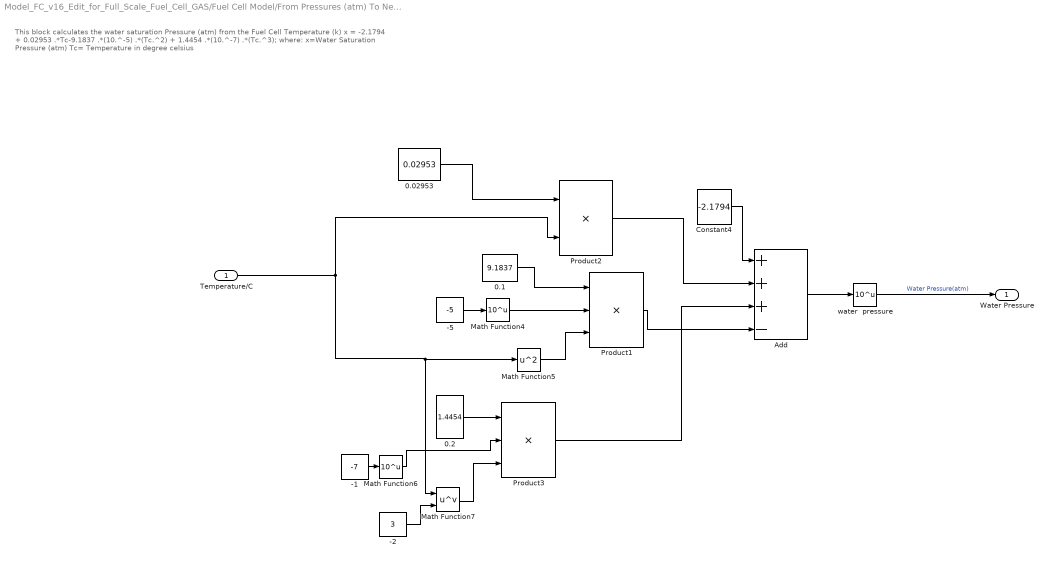
== system Model_FC_v16_Edit_for_Full_Scale_Fuel_Cell_GAS/Fuel Cell Model/From Pressures (atm) To Nernest Voltage (V)/From Absolute Pressure (atm) To Partial Pressures (atm)/Water Pressure output ==
  note: This block calculates the water saturation Pressure (atm) from the Fuel Cell Temperature (k)
      | x = -2.1794 + 0.02953 .*Tc-9.1837 .*(10.^-5) .*(Tc.^2) + 1.4454 .*(10.^-7) .*(Tc.^3);
      | where: x=Water Saturation Pressure (atm)
      | Tc= Temperature in degree celsius
  Temperature/C : Inport
  -1 : Constant  Value=-7
  -2 : Constant  Value=3
  -5 : Constant  Value=-5
  0.02953 : Constant  Value=0.02953
  0.1 : Constant  Value=9.1837
  0.2 : Constant  Value=1.4454
  Add : Sum  Inputs=+++-
  Constant4 : Constant  Value=-2.1794
  Math Function4 : Math  Operator=10^u  SaturateOnIntegerOverflow=on
  Math Function5 : Math  Operator=square  SaturateOnIntegerOverflow=on
  Math Function6 : Math  Operator=10^u  SaturateOnIntegerOverflow=on
  Math Function7 : Math  Operator=pow  SaturateOnIntegerOverflow=on
  Product1 : Product  Inputs=3
  Product2 : Product
  Product3 : Product  Inputs=3
  "water  pressure " : Math  Operator=10^u  SaturateOnIntegerOverflow=on
  Water Pressure : Outport
  wires:
  Add/1 -> "water  pressure "/1
  0.2/1 -> Product3/1
  Math Function7/1 -> Product3/3
  "water  pressure "/1 -> Water Pressure/1  "Water Pressure(atm)"
  0.02953/1 -> Product2/1
  0.1/1 -> Product1/1
  -5/1 -> Math Function4/1
  Math Function4/1 -> Product1/2
  -1/1 -> Math Function6/1
  Temperature/C/1 -> Product2/2, Math Function5/1, Math Function7/1
  Math Function5/1 -> Product1/3
  -2/1 -> Math Function7/2
  Product2/1 -> Add/2
  Product3/1 -> Add/3
  Math Function6/1 -> Product3/2
  Constant4/1 -> Add/1
  Product1/1 -> Add/4

== system Model_FC_v16_Edit_for_Full_Scale_Fuel_Cell_GAS/Fuel Cell Model/From Pressures (atm) To Nernest Voltage (V)/From Partial Pressures (atm) To Nernest Voltage (V)/IF Function ==
  In1 : Inport
  Constant1 : Constant
  If : If
  If Action Subsystem : Subsystem  TreatAsAtomicUnit=on
  If Action Subsystem1 : Subsystem  TreatAsAtomicUnit=on
  Merge : Merge
  Out1 : Outport
  wires:
  Constant1/1 -> If Action Subsystem1/1(In1)
  If Action Subsystem1/1(Out1) -> Merge/2
  If/1 -> If Action Subsystem/Action
  If/2 -> If Action Subsystem1/Action
  In1/1 -> If Action Subsystem/1(In1), If/1
  Merge/1 -> Out1/1
  If Action Subsystem/1(Out1) -> Merge/1

== system Model_FC_v16_Edit_for_Full_Scale_Fuel_Cell_GAS/Fuel Cell Model/ From Current Density (A//cm^2) To Overvoltages (V)/Concentration Overvoltage/IF Function/If Action Subsystem ==
  In1 : Inport
  Action Port : ActionPort  ActionType=then
  Math Function1 : Math  Operator=log  OutputSignalType=real  SaturateOnIntegerOverflow=on
  Out1 : Outport
  wires:
  In1/1 -> Math Function1/1
  Math Function1/1 -> Out1/1

== system Model_FC_v16_Edit_for_Full_Scale_Fuel_Cell_GAS/Fuel Cell Model/ From Current Density (A//cm^2) To Overvoltages (V)/Concentration Overvoltage/IF Function/If Action Subsystem1 ==
  Action Port : ActionPort  ActionType=else
  Constant1 : Constant  Value=0
  Out1 : Outport
  wires:
  Constant1/1 -> Out1/1

== system Model_FC_v16_Edit_for_Full_Scale_Fuel_Cell_GAS/Fuel Cell Model/From Pressures (atm) To Nernest Voltage (V)/From Partial Pressures (atm) To Nernest Voltage (V)/IF Function/If Action Subsystem ==
  In1 : Inport
  Action Port : ActionPort  ActionType=then
  Out1 : Outport
  wires:
  In1/1 -> Out1/1

== system Model_FC_v16_Edit_for_Full_Scale_Fuel_Cell_GAS/Fuel Cell Model/From Pressures (atm) To Nernest Voltage (V)/From Partial Pressures (atm) To Nernest Voltage (V)/IF Function/If Action Subsystem1 ==
  In1 : Inport
  Action Port : ActionPort  ActionType=else
  Out1 : Outport
  wires:
  In1/1 -> Out1/1
